simulink model "DFIG_FILTER"  (R2023a)
settings: Solver=ode23t  StartTime=0.0  StopTime=25  MaxStep=1e-6  RelTol=1e-3
model workspace (MAT data in the model file):
  Ts_phasor = 10
undefined symbols (not defined in the file): Base_Power, D1, Delta, F, find_system, Fnom, gcbh, H, ILd_init, ILq_init, Imax_grid_conv, Init, j, Ki_dc_reg, Ki_grid_side_cur_reg, Ki_power_reg, Ki_Q, Ki_rotor_side_cur_reg, Ki_volt_reg, Kp_dc_reg, Kp_grid_side_cur_reg, Kp_power_reg, Kp_Q, Kp_rotor_side_cur_reg, Kp_volt_reg, L_RL, Llr, Lls, p, Pnom, power_A, power_B, power_D, R_RL, Rr, Rs, speed_A, speed_B, speed_C, speed_D, sps_rtmsupport, Vcontrol, Vnom, Wind_On
libraries: spsPower3phPhasorLib x9, spsOnDelayLib x9, spsThreePhaseVIMeasurementLib x8, simulink_extras x5, spsRMSLib x4, spsControlledCurrentSourceLib x4, spsGroundLib x3, spsSeriesRLCBranchLib x2, spsThreePhaseSeriesRLCBranchLib x2, spspowerguiLib x2, spsThreePhasePISectionLineLib x2, spsThreePhaseTransformerTwoWindingsLib x2
(part 2 of 6)

== system DFIG_FILTER/MODEL (PHASER)/Wind turbine Data acquisition2 ==
  Constant : Constant  Value=0
  Gain3 : Gain  Gain=1/3  SaturateOnIntegerOverflow=on  OutDataTypeStr=Inherit: Same as input  ParamDataTypeStr=Inherit: Same as input
  Gain4 : Gain  Gain=1/3  SaturateOnIntegerOverflow=on  OutDataTypeStr=Inherit: Same as input  ParamDataTypeStr=Inherit: Same as input
  MW : Gain  Gain=-1/1e6  SaturateOnIntegerOverflow=on  OutDataTypeStr=Inherit: Same as input  ParamDataTypeStr=Inherit: Same as input
  MW1 : Gain  Gain=-1/1e6  SaturateOnIntegerOverflow=on  OutDataTypeStr=Inherit: Same as input  ParamDataTypeStr=Inherit: Same as input
  Mean Value1 : Subsystem  mask(Mean value){Period=1/60}
      mask prompts: Period "Averaging period (s):"
      mask help: This block uses the running window averaging technique to compute the mean value of the input signal over the specified period.
  Mean Value2 : Subsystem  mask(Mean value){Period=1/60}
      mask prompts: Period "Averaging period (s):"
      mask help: This block uses the running window averaging technique to compute the mean value of the input signal over the specified period.
  "Power (3ph, Phasor)" : spsPower3phPhasorLib/Power (3ph, Phasor)
  Sum : Sum  Inputs=1  InputSameDT=on  SaturateOnIntegerOverflow=on  OutDataTypeStr=Inherit: Same as first input
  Sum1 : Sum  Inputs=1  InputSameDT=on  SaturateOnIntegerOverflow=on  OutDataTypeStr=Inherit: Same as first input
  abc_to_pos : Gain  Gain=[1 exp(j*2*pi/3) exp(-j*2*pi/3)]  SaturateOnIntegerOverflow=on  OutDataTypeStr=Inherit: Same as input  ParamDataTypeStr=Inherit: Same as input
  abc_to_pos1 : Gain  Gain=[1 exp(j*2*pi/3) exp(-j*2*pi/3)]  SaturateOnIntegerOverflow=on  OutDataTypeStr=Inherit: Same as input  ParamDataTypeStr=Inherit: Same as input
  "magnitude positive seq. " : Subsystem
  magnitude positivie seq : Subsystem
  pu->A : Gain  Gain=(6*1.5e6/0.9)/sqrt(3)/575*sqrt(2)  SaturateOnIntegerOverflow=on  OutDataTypeStr=Inherit: Same as input  ParamDataTypeStr=Inherit: Same as input
  pu->V : Gain  Gain=575*sqrt(2)/sqrt(3)  SaturateOnIntegerOverflow=on  OutDataTypeStr=Inherit: Same as input  ParamDataTypeStr=Inherit: Same as input
  Vabc_BFF : Outport  VectorParamsAs1DForOutWhenUnconnected=off
  Iabc_BFF : Outport  Port=2  VectorParamsAs1DForOutWhenUnconnected=off
  P_mean : Outport  Port=3  VectorParamsAs1DForOutWhenUnconnected=off
  Q_mean : Outport  Port=4  VectorParamsAs1DForOutWhenUnconnected=off
  wires:
  [Iabc_BFF] -> abc_to_pos1/1, pu->A/1
  [Vabc_BFF] -> pu->V/1, abc_to_pos/1
  pu->A/1 -> "Power (3ph, Phasor)"/2
  pu->V/1 -> "Power (3ph, Phasor)"/1
  MW/1 -> Mean Value1/1(In)
  MW1/1 -> Mean Value2/1(In)
  "magnitude positive seq. "/1(Out1) -> Iabc_BFF/1
  magnitude positivie seq/1(Out1) -> Vabc_BFF/1
  abc_to_pos/1 -> Sum/1
  Sum/1 -> Gain3/1
  Sum1/1 -> Gain4/1
  Gain3/1 -> magnitude positivie seq/1(In1)
  abc_to_pos1/1 -> Sum1/1
  Gain4/1 -> "magnitude positive seq. "/1(In1)
  Mean Value1/1(Mean) -> P_mean/1
  Mean Value2/1(Mean) -> Q_mean/1
  Constant/1 -> Mean Value1/2(Init), Mean Value2/2(Init)
  "Power (3ph, Phasor)"/1 -> MW/1
  "Power (3ph, Phasor)"/2 -> MW1/1

== system DFIG_FILTER/MODEL (PHASER)/Wind turbine Data acquisition3 ==
  Constant : Constant  Value=0
  Gain3 : Gain  Gain=1/3  SaturateOnIntegerOverflow=on  OutDataTypeStr=Inherit: Same as input  ParamDataTypeStr=Inherit: Same as input
  Gain4 : Gain  Gain=1/3  SaturateOnIntegerOverflow=on  OutDataTypeStr=Inherit: Same as input  ParamDataTypeStr=Inherit: Same as input
  MW : Gain  Gain=-1/1e6  SaturateOnIntegerOverflow=on  OutDataTypeStr=Inherit: Same as input  ParamDataTypeStr=Inherit: Same as input
  MW1 : Gain  Gain=-1/1e6  SaturateOnIntegerOverflow=on  OutDataTypeStr=Inherit: Same as input  ParamDataTypeStr=Inherit: Same as input
  Mean Value1 : Subsystem  mask(Mean value){Period=1/60}
      mask prompts: Period "Averaging period (s):"
      mask help: This block uses the running window averaging technique to compute the mean value of the input signal over the specified period.
  Mean Value2 : Subsystem  mask(Mean value){Period=1/60}
      mask prompts: Period "Averaging period (s):"
      mask help: This block uses the running window averaging technique to compute the mean value of the input signal over the specified period.
  "Power (3ph, Phasor)" : spsPower3phPhasorLib/Power (3ph, Phasor)
  Sum : Sum  Inputs=1  InputSameDT=on  SaturateOnIntegerOverflow=on  OutDataTypeStr=Inherit: Same as first input
  Sum1 : Sum  Inputs=1  InputSameDT=on  SaturateOnIntegerOverflow=on  OutDataTypeStr=Inherit: Same as first input
  abc_to_pos : Gain  Gain=[1 exp(j*2*pi/3) exp(-j*2*pi/3)]  SaturateOnIntegerOverflow=on  OutDataTypeStr=Inherit: Same as input  ParamDataTypeStr=Inherit: Same as input
  abc_to_pos1 : Gain  Gain=[1 exp(j*2*pi/3) exp(-j*2*pi/3)]  SaturateOnIntegerOverflow=on  OutDataTypeStr=Inherit: Same as input  ParamDataTypeStr=Inherit: Same as input
  "magnitude positive seq. " : Subsystem
  magnitude positivie seq : Subsystem
  pu->A : Gain  Gain=(6*1.5e6/0.9)/sqrt(3)/575*sqrt(2)  SaturateOnIntegerOverflow=on  OutDataTypeStr=Inherit: Same as input  ParamDataTypeStr=Inherit: Same as input
  pu->V : Gain  Gain=575*sqrt(2)/sqrt(3)  SaturateOnIntegerOverflow=on  OutDataTypeStr=Inherit: Same as input  ParamDataTypeStr=Inherit: Same as input
  Vabc_BFF : Outport  VectorParamsAs1DForOutWhenUnconnected=off
  Iabc_BFF : Outport  Port=2  VectorParamsAs1DForOutWhenUnconnected=off
  P_mean : Outport  Port=3  VectorParamsAs1DForOutWhenUnconnected=off
  Q_mean : Outport  Port=4  VectorParamsAs1DForOutWhenUnconnected=off
  wires:
  [Iabc_BFF] -> abc_to_pos1/1, pu->A/1
  [Vabc_BFF] -> pu->V/1, abc_to_pos/1
  pu->A/1 -> "Power (3ph, Phasor)"/2
  pu->V/1 -> "Power (3ph, Phasor)"/1
  MW/1 -> Mean Value1/1(In)
  MW1/1 -> Mean Value2/1(In)
  "magnitude positive seq. "/1(Out1) -> Iabc_BFF/1
  magnitude positivie seq/1(Out1) -> Vabc_BFF/1
  abc_to_pos/1 -> Sum/1
  Sum/1 -> Gain3/1
  Sum1/1 -> Gain4/1
  Gain3/1 -> magnitude positivie seq/1(In1)
  abc_to_pos1/1 -> Sum1/1
  Gain4/1 -> "magnitude positive seq. "/1(In1)
  Mean Value1/1(Mean) -> P_mean/1
  Mean Value2/1(Mean) -> Q_mean/1
  Constant/1 -> Mean Value1/2(Init), Mean Value2/2(Init)
  "Power (3ph, Phasor)"/1 -> MW/1
  "Power (3ph, Phasor)"/2 -> MW1/1

== system DFIG_FILTER/MODEL (PHASER)/Wind turbine Data acquisition4 ==
  Constant : Constant  Value=0
  Gain3 : Gain  Gain=1/3  SaturateOnIntegerOverflow=on  OutDataTypeStr=Inherit: Same as input  ParamDataTypeStr=Inherit: Same as input
  Gain4 : Gain  Gain=1/3  SaturateOnIntegerOverflow=on  OutDataTypeStr=Inherit: Same as input  ParamDataTypeStr=Inherit: Same as input
  MW : Gain  Gain=-1/1e6  SaturateOnIntegerOverflow=on  OutDataTypeStr=Inherit: Same as input  ParamDataTypeStr=Inherit: Same as input
  MW1 : Gain  Gain=-1/1e6  SaturateOnIntegerOverflow=on  OutDataTypeStr=Inherit: Same as input  ParamDataTypeStr=Inherit: Same as input
  Mean Value1 : Subsystem  mask(Mean value){Period=1/60}
      mask prompts: Period "Averaging period (s):"
      mask help: This block uses the running window averaging technique to compute the mean value of the input signal over the specified period.
  Mean Value2 : Subsystem  mask(Mean value){Period=1/60}
      mask prompts: Period "Averaging period (s):"
      mask help: This block uses the running window averaging technique to compute the mean value of the input signal over the specified period.
  "Power (3ph, Phasor)" : spsPower3phPhasorLib/Power (3ph, Phasor)
  Sum : Sum  Inputs=1  InputSameDT=on  SaturateOnIntegerOverflow=on  OutDataTypeStr=Inherit: Same as first input
  Sum1 : Sum  Inputs=1  InputSameDT=on  SaturateOnIntegerOverflow=on  OutDataTypeStr=Inherit: Same as first input
  abc_to_pos : Gain  Gain=[1 exp(j*2*pi/3) exp(-j*2*pi/3)]  SaturateOnIntegerOverflow=on  OutDataTypeStr=Inherit: Same as input  ParamDataTypeStr=Inherit: Same as input
  abc_to_pos1 : Gain  Gain=[1 exp(j*2*pi/3) exp(-j*2*pi/3)]  SaturateOnIntegerOverflow=on  OutDataTypeStr=Inherit: Same as input  ParamDataTypeStr=Inherit: Same as input
  "magnitude positive seq. " : Subsystem
  magnitude positivie seq : Subsystem
  pu->A : Gain  Gain=(6*1.5e6/0.9)/sqrt(3)/575*sqrt(2)  SaturateOnIntegerOverflow=on  OutDataTypeStr=Inherit: Same as input  ParamDataTypeStr=Inherit: Same as input
  pu->V : Gain  Gain=575*sqrt(2)/sqrt(3)  SaturateOnIntegerOverflow=on  OutDataTypeStr=Inherit: Same as input  ParamDataTypeStr=Inherit: Same as input
  Vabc_BAF : Outport  VectorParamsAs1DForOutWhenUnconnected=off
  Iabc_BAF : Outport  Port=2  VectorParamsAs1DForOutWhenUnconnected=off
  P_mean : Outport  Port=3  VectorParamsAs1DForOutWhenUnconnected=off
  Q_mean : Outport  Port=4  VectorParamsAs1DForOutWhenUnconnected=off
  wires:
  [Iabc_BAF] -> abc_to_pos1/1, pu->A/1
  [Vabc_BAF] -> pu->V/1, abc_to_pos/1
  pu->A/1 -> "Power (3ph, Phasor)"/2
  pu->V/1 -> "Power (3ph, Phasor)"/1
  MW/1 -> Mean Value1/1(In)
  MW1/1 -> Mean Value2/1(In)
  "magnitude positive seq. "/1(Out1) -> Iabc_BAF/1
  magnitude positivie seq/1(Out1) -> Vabc_BAF/1
  abc_to_pos/1 -> Sum/1
  Sum/1 -> Gain3/1
  Sum1/1 -> Gain4/1
  Gain3/1 -> magnitude positivie seq/1(In1)
  abc_to_pos1/1 -> Sum1/1
  Gain4/1 -> "magnitude positive seq. "/1(In1)
  Mean Value1/1(Mean) -> P_mean/1
  Mean Value2/1(Mean) -> Q_mean/1
  Constant/1 -> Mean Value1/2(Init), Mean Value2/2(Init)
  "Power (3ph, Phasor)"/1 -> MW/1
  "Power (3ph, Phasor)"/2 -> MW1/1

== system DFIG_FILTER/MODEL (PHASER)/Wind turbine Data acquisition5 ==
  Constant : Constant  Value=0
  Gain3 : Gain  Gain=1/3  SaturateOnIntegerOverflow=on  OutDataTypeStr=Inherit: Same as input  ParamDataTypeStr=Inherit: Same as input
  Gain4 : Gain  Gain=1/3  SaturateOnIntegerOverflow=on  OutDataTypeStr=Inherit: Same as input  ParamDataTypeStr=Inherit: Same as input
  MW : Gain  Gain=-1/1e6  SaturateOnIntegerOverflow=on  OutDataTypeStr=Inherit: Same as input  ParamDataTypeStr=Inherit: Same as input
  MW1 : Gain  Gain=-1/1e6  SaturateOnIntegerOverflow=on  OutDataTypeStr=Inherit: Same as input  ParamDataTypeStr=Inherit: Same as input
  Mean Value1 : Subsystem  mask(Mean value){Period=1/60}
      mask prompts: Period "Averaging period (s):"
      mask help: This block uses the running window averaging technique to compute the mean value of the input signal over the specified period.
  Mean Value2 : Subsystem  mask(Mean value){Period=1/60}
      mask prompts: Period "Averaging period (s):"
      mask help: This block uses the running window averaging technique to compute the mean value of the input signal over the specified period.
  "Power (3ph, Phasor)" : spsPower3phPhasorLib/Power (3ph, Phasor)
  Sum : Sum  Inputs=1  InputSameDT=on  SaturateOnIntegerOverflow=on  OutDataTypeStr=Inherit: Same as first input
  Sum1 : Sum  Inputs=1  InputSameDT=on  SaturateOnIntegerOverflow=on  OutDataTypeStr=Inherit: Same as first input
  abc_to_pos : Gain  Gain=[1 exp(j*2*pi/3) exp(-j*2*pi/3)]  SaturateOnIntegerOverflow=on  OutDataTypeStr=Inherit: Same as input  ParamDataTypeStr=Inherit: Same as input
  abc_to_pos1 : Gain  Gain=[1 exp(j*2*pi/3) exp(-j*2*pi/3)]  SaturateOnIntegerOverflow=on  OutDataTypeStr=Inherit: Same as input  ParamDataTypeStr=Inherit: Same as input
  "magnitude positive seq. " : Subsystem
  magnitude positivie seq : Subsystem
  pu->A : Gain  Gain=(6*1.5e6/0.9)/sqrt(3)/575*sqrt(2)  SaturateOnIntegerOverflow=on  OutDataTypeStr=Inherit: Same as input  ParamDataTypeStr=Inherit: Same as input
  pu->V : Gain  Gain=575*sqrt(2)/sqrt(3)  SaturateOnIntegerOverflow=on  OutDataTypeStr=Inherit: Same as input  ParamDataTypeStr=Inherit: Same as input
  Vabc_BAF : Outport  VectorParamsAs1DForOutWhenUnconnected=off
  Iabc_BAF : Outport  Port=2  VectorParamsAs1DForOutWhenUnconnected=off
  P_mean : Outport  Port=3  VectorParamsAs1DForOutWhenUnconnected=off
  Q_mean : Outport  Port=4  VectorParamsAs1DForOutWhenUnconnected=off
  wires:
  [Vabc_B575] -> abc_to_pos1/1, pu->A/1
  [Vabc_B575] -> pu->V/1, abc_to_pos/1
  pu->A/1 -> "Power (3ph, Phasor)"/2
  pu->V/1 -> "Power (3ph, Phasor)"/1
  MW/1 -> Mean Value1/1(In)
  MW1/1 -> Mean Value2/1(In)
  "magnitude positive seq. "/1(Out1) -> Iabc_BAF/1
  magnitude positivie seq/1(Out1) -> Vabc_BAF/1
  abc_to_pos/1 -> Sum/1
  Sum/1 -> Gain3/1
  Sum1/1 -> Gain4/1
  Gain3/1 -> magnitude positivie seq/1(In1)
  abc_to_pos1/1 -> Sum1/1
  Gain4/1 -> "magnitude positive seq. "/1(In1)
  Mean Value1/1(Mean) -> P_mean/1
  Mean Value2/1(Mean) -> Q_mean/1
  Constant/1 -> Mean Value1/2(Init), Mean Value2/2(Init)
  "Power (3ph, Phasor)"/1 -> MW/1
  "Power (3ph, Phasor)"/2 -> MW1/1

== system DFIG_FILTER/FILTER (DISCRETE) /controller1/WMPID ==
  In1 : Inport  PortDimensions=3
  Cast To Double : DataTypeConversion  OutDataTypeStr=double  SaturateOnIntegerOverflow=off  RndMeth=Floor
  Cast To Double1 : DataTypeConversion  OutDataTypeStr=double  SaturateOnIntegerOverflow=off  RndMeth=Floor
  Derivative : Derivative
  Integrator : Integrator
  Kd : Gain
  Ke : Gain
  Ki : Gain  Gain=2
  Kp : Gain  Gain=25
  Product1 : Product
  Sum7 : Sum  Inputs=|+++
  Sum8 : Sum  Inputs=|++
  Out1 : Outport  PortDimensions=3
  wires:
  In1/1 -> Kp/1, Product1/2, Product1/1, Derivative/1, Ki/1
  Sum8/1 -> Out1/1
  Integrator/1 -> Sum7/2
  Derivative/1 -> Kd/1
  Product1/1 -> Ke/1
  Kd/1 -> Sum7/3
  Ki/1 -> Integrator/1
  Kp/1 -> Sum7/1
  Ke/1 -> Cast To Double/1
  Cast To Double/1 -> Sum8/1
  Sum7/1 -> Cast To Double1/1
  Cast To Double1/1 -> Sum8/2

== system DFIG_FILTER/MODEL (PHASER)/Grid Data acquisition/Mean Value1 ==
  note: Mean value
  In : Inport
  Init : Inport  Port=2
  Gain : Gain  Gain=1/Period  SaturateOnIntegerOverflow=on  OutDataTypeStr=Inherit: Same as input  ParamDataTypeStr=Inherit: Same as input
  Step : Step  Time=Period+eps  SampleTime=0
  Sum : Sum  Inputs=+-  InputSameDT=on  SaturateOnIntegerOverflow=on  OutDataTypeStr=Inherit: Same as first input
  Switch : Switch  Threshold=0.5  InputSameDT=off
  Transport Delay : TransportDelay  DelayTime=Period
  integrator : Integrator
  Mean : Outport  VectorParamsAs1DForOutWhenUnconnected=off
  wires:
  Transport Delay/1 -> Sum/2
  integrator/1 -> Transport Delay/1, Sum/1
  In/1 -> integrator/1
  Sum/1 -> Gain/1
  Gain/1 -> Switch/1
  Switch/1 -> Mean/1
  Step/1 -> Switch/2
  Init/1 -> Switch/3

== system DFIG_FILTER/MODEL (PHASER)/Grid Data acquisition/Mean Value2 ==
  note: Mean value
  In : Inport
  Init : Inport  Port=2
  Gain : Gain  Gain=1/Period  SaturateOnIntegerOverflow=on  OutDataTypeStr=Inherit: Same as input  ParamDataTypeStr=Inherit: Same as input
  Step : Step  Time=Period+eps  SampleTime=0
  Sum : Sum  Inputs=+-  InputSameDT=on  SaturateOnIntegerOverflow=on  OutDataTypeStr=Inherit: Same as first input
  Switch : Switch  Threshold=0.5  InputSameDT=off
  Transport Delay : TransportDelay  DelayTime=Period
  integrator : Integrator
  Mean : Outport  VectorParamsAs1DForOutWhenUnconnected=off
  wires:
  Init/1 -> Switch/3
  Step/1 -> Switch/2
  Switch/1 -> Mean/1
  Gain/1 -> Switch/1
  Sum/1 -> Gain/1
  In/1 -> integrator/1
  integrator/1 -> Sum/1, Transport Delay/1
  Transport Delay/1 -> Sum/2

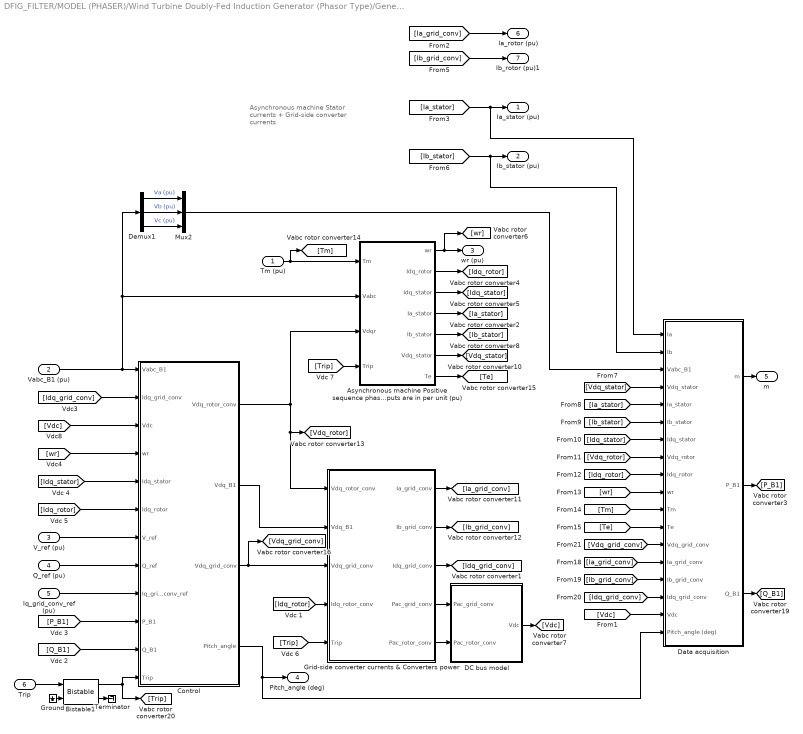
== system DFIG_FILTER/MODEL (PHASER)/Wind Turbine Doubly-Fed Induction Generator (Phasor Type)/Generator & Converters ==
  note: Asynchronous machine
      | Stator currents
      | +
      | Grid-side converter
      | currents
  Tm (pu) : Inport
  Vabc_B1 (pu) : Inport  Port=2
  V_ref (pu) : Inport  Port=3
  Q_ref (pu) : Inport  Port=4
  Iq_grid_conv_ref (pu) : Inport  Port=5
  Trip : Inport  Port=6
  Asynchronous machine Positive sequence phasor model Inputs and outputs are in per unit (pu) : Subsystem  mask(Asynchronous Machine Model){nom=[ Pnom Vnom Fnom ], sta=[ Rs Lls], rot=[ Rr Llr], Lm=Lm, mec=[H F p], ini=init}
      mask prompts: nom "Nom. power,L-L volt. and freq. [ Pn(VA),Vn(Vrms),fn(Hz) ]:"; sta "Stator [ Rs,Lls (pu) ]:"; rot "Rotor [ Rr',Llr' (pu) ]:"; Lm "Magnetizing inductance Lm (pu):"; mec "Inertia constant,friction factor and pairs of poles [ H(s)  F(pu)  p() ]:"; ini "Initial conditions [s()  th(deg)  Is(pu)  ph_Is(deg)  Ir(pu)  ph_Ir(deg)]:"
      mask help: Implements a three-phase asynchronous machine (wound rotor) modelled in the dq stator reference frame. Stator and rotor windings are connected in wye to an internal neutral point.
      mask init:
      | %Initializes the Asynchronous Machine block before simulation.
      | 
      | % Base angular frequency
      | web=nom(3)*2*pi;
      | 
      | Rs=sta(1); Lls=sta(2);		% stator resistance and leakage inductance
      | Rr=rot(1); Llr=rot(2);		% rotor resistance and leakage inductance
      | Lm=Lm(1);			        % mutual inductance
      | H=mec(1); F=mec(2); p=mec(3);	% inertia, friction and pole pairs
      | s=ini(1);			% initial slip
      | wmo=1-s;			% initial speed
      | tho=ini(2)*pi/180;		% initial rotor angle
      | 
      | iso_mag=ini(3); iso_ph=ini(4)*pi/180; % init. stator current, phase A
      | iro_mag=ini(5); iro_ph=ini(6)*pi/180; % init. rotor current, phase A
      | 
      | % conversion of initial stator and rotor currents from polar to rectangular
      | % coordinates
      | [isdo,isqo]=pol2cart(iso_ph,iso_mag);
      | [irdo,irqo]=pol2cart(iro_ph,iro_mag);
      | 
      | % Initial fluxes (pu): inductances in pu, currents in pu
      | phisqo=((Lls+Lm)*isqo+Lm*irqo);
      | phisdo=((Lls+Lm)*isdo+Lm*irdo);
      | phirqo=((Llr+Lm)*irqo+Lm*isqo);
      | phirdo=((Llr+Lm)*irdo+Lm*isdo);
      | 
      | % Other inductances -------------------------------------------------------
      | 
      | Laq=1/(1/Lm+1/Lls+1/Llr);
      | Lad=Laq;
      mask Help: First 3 inputs: Stator terminals = phases a, b and c; 4th input: Simulink signal = Mechanical torque applied to the shaft (pu, >0 for motor mode, <0 for generator mode); First 3 outputs: Rotor terminals = phases a, b and c; 4th output: Simulink measurement output = vector (20x1) containing the following (all currents flowing into the machine): [1-3] : Rotor line currents ira, irb and irc; [4-5] : Rotor currents iqr and idr; [6-7] : Rotor fluxes phiqr and  phidr; [8-9] : Rotor voltages vqr and vdr; [10-12] : Stator line currents isa, isb, isc; [13-14] : Stator currents iqs and ids; [15-16] : Stator fluxes phiqs and  phids; [17-18] : Stator voltages vqs and vds; [19] : Rotor speed wm; [20 ]: Electromagnetic torque Te. Units of output measurement depend on checkbox in block's dialog box.
  Bistable1 : spsBistableLib/Bistable  Qpriority=Set  ic=0  Ts=0
      settings: LibrarySourceBlock=sps_lib/Control/Bistable
  Control : Subsystem
  DC bus model : Subsystem  mask(DC bus model){Pnom=Pnom, C=capacitor, Vdc_Init=Vdc_nom}
      mask prompts: Pnom "Nominal power (W):"; C "Capacitor (F):"; Vdc_Init "Initial voltage (V):"
  Data acquisition : Subsystem
  Demux1 : Demux  Outputs=3
      settings: DisplayOption=none
  Grid-side converter currents & Converters power : Subsystem
  Ground : Ground
  Mux2 : Mux  Inputs=3
  Terminator : Terminator
  Ia_stator (pu) : Outport  VectorParamsAs1DForOutWhenUnconnected=off
  Ib_stator (pu) : Outport  Port=2  VectorParamsAs1DForOutWhenUnconnected=off
  wr (pu) : Outport  Port=3  VectorParamsAs1DForOutWhenUnconnected=off
  Pitch_angle (deg) : Outport  Port=4  VectorParamsAs1DForOutWhenUnconnected=off
  m : Outport  Port=5  VectorParamsAs1DForOutWhenUnconnected=off
  Ia_rotor (pu) : Outport  Port=6  VectorParamsAs1DForOutWhenUnconnected=off
  Ib_rotor (pu)1 : Outport  Port=7  VectorParamsAs1DForOutWhenUnconnected=off
  wires:
  DC bus model/1(Vdc) -> [Vdc]
  [Idq_rotor] -> Control/6(Idq_rotor)
  [Idq_stator] -> Control/5(Idq_stator)
  [Vdc] -> Control/3(Vdc)
  [wr] -> Control/4(wr)
  Control/3(Vdq_grid_conv) -> Grid-side converter currents & Converters power/3(Vdq_grid_conv), [Vdq_grid_conv]
  Control/1(Vdq_rotor_conv) -> Asynchronous machine Positive sequence phasor model Inputs and outputs are in per unit (pu)/3("Vdqr "), Grid-side converter currents & Converters power/1(Vdq_rotor_conv), [Vdq_rotor]
  Control/2(Vdq_B1) -> Grid-side converter currents & Converters power/2(Vdq_B1)
  Grid-side converter currents & Converters power/3(Idq_grid_conv) -> [Idq_grid_conv]
  [Idq_grid_conv] -> Control/2(Idq_grid_conv)
  Asynchronous machine Positive sequence phasor model Inputs and outputs are in per unit (pu)/3(Idq_stator) -> [Idq_stator]
  Asynchronous machine Positive sequence phasor model Inputs and outputs are in per unit (pu)/2(Idq_rotor) -> [Idq_rotor]
  Tm (pu)/1 -> Asynchronous machine Positive sequence phasor model Inputs and outputs are in per unit (pu)/1(Tm), [Tm]
  Asynchronous machine Positive sequence phasor model Inputs and outputs are in per unit (pu)/5(Ib_stator) -> [Ib_stator]
  Asynchronous machine Positive sequence phasor model Inputs and outputs are in per unit (pu)/4(Ia_stator) -> [Ia_stator]
  [Idq_rotor] -> Grid-side converter currents & Converters power/4(Idq_rotor_conv)
  Grid-side converter currents & Converters power/4(Pac_grid_conv) -> DC bus model/1(Pac_grid_conv)
  Grid-side converter currents & Converters power/5(Pac_rotor_conv) -> DC bus model/2(Pac_rotor_conv)
  Vabc_B1 (pu)/1 -> Control/1(Vabc_B1), Asynchronous machine Positive sequence phasor model Inputs and outputs are in per unit (pu)/2(Vabc), Demux1/1
  [Ia_stator] -> Ia_stator (pu)/1, Data acquisition/1(Ia)
  [Ib_stator] -> Ib_stator (pu)/1, Data acquisition/2(Ib)
  Asynchronous machine Positive sequence phasor model Inputs and outputs are in per unit (pu)/1(wr) -> wr (pu)/1, [wr]
  Asynchronous machine Positive sequence phasor model Inputs and outputs are in per unit (pu)/6(Vdq_stator) -> [Vdq_stator]
  Grid-side converter currents & Converters power/1(Ia_grid_conv) -> [Ia_grid_conv]
  Grid-side converter currents & Converters power/2(Ib_grid_conv) -> [Ib_grid_conv]
  [Ia_grid_conv] -> Ia_rotor (pu)/1
  [Ib_grid_conv] -> Ib_rotor (pu)1/1
  Asynchronous machine Positive sequence phasor model Inputs and outputs are in per unit (pu)/7(Te) -> [Te]
  [Idq_grid_conv] -> Data acquisition/16(Idq_grid_conv)
  [Ib_grid_conv] -> Data acquisition/15(Ib_grid_conv)
  [Ia_grid_conv] -> Data acquisition/14(Ia_grid_conv)
  [Vdq_grid_conv] -> Data acquisition/13(Vdq_grid_conv)
  [Te] -> Data acquisition/12(Te)
  [Tm] -> Data acquisition/11(Tm)
  [wr] -> Data acquisition/10(wr)
  [Idq_rotor] -> Data acquisition/9(Idq_rotor)
  [Vdq_rotor] -> Data acquisition/8(Vdq_rotor)
  [Idq_stator] -> Data acquisition/7(Idq_stator)
  [Ib_stator] -> Data acquisition/6(Ib_stator)
  [Ia_stator] -> Data acquisition/5(Ia_stator)
  [Vdq_stator] -> Data acquisition/4(Vdq_stator)
  Data acquisition/1(m) -> m/1
  [Vdc] -> Data acquisition/17(Vdc)
  Demux1/1 -> Mux2/1  "Va (pu)"
  Demux1/2 -> Mux2/2  "Vb (pu)"
  Mux2/1 -> Data acquisition/3(Vabc_B1)
  Demux1/3 -> Mux2/3  "Vc (pu)"
  Data acquisition/3(Q_B1) -> [Q_B1]
  Q_ref (pu)/1 -> Control/8(Q_ref)
  Iq_grid_conv_ref (pu)/1 -> Control/9(Iq_grid_conv_ref)
  Data acquisition/2(P_B1) -> [P_B1]
  [P_B1] -> Control/10(P_B1)
  [Q_B1] -> Control/11(Q_B1)
  V_ref (pu)/1 -> Control/7(V_ref)
  [Trip] -> Grid-side converter currents & Converters power/5(Trip)
  [Trip] -> Asynchronous machine Positive sequence phasor model Inputs and outputs are in per unit (pu)/4(Trip)
  Trip/1 -> Bistable1/1
  Bistable1/2 -> Terminator/1
  Ground/1 -> Bistable1/2
  Bistable1/1 -> [Trip], Control/12(Trip)
  Control/4(Pitch_angle) -> Data acquisition/18(Pitch_angle (deg)), Pitch_angle (deg)/1

== system DFIG_FILTER/MODEL (PHASER)/Wind Turbine Protection/Protection System ==
  Vabc (pu) : Inport  PortDimensions=3
  Iabc (pu) : Inport  Port=2  PortDimensions=3
  Vdc (V) : Inport  Port=3  PortDimensions=1
  Reset : Inport  Port=4  PortDimensions=1
  Speed (pu) : Inport  Port=5  PortDimensions=1
  AC Current Protection : Subsystem
  AC Voltage Protection : Subsystem
  Bistable1 : spsBistableLib/Bistable  Qpriority=Set  ic=0  Ts=0
  Clock : Clock
  Constant : Constant  Value=Delay_Protection
  DC Voltage Protection : Subsystem
  Decoding : Subsystem
  Encoding : Subsystem
  Logical Operator : Logic  Operator=OR  Inputs=10  AllPortsSameDT=off
  Logical Operator1 : Logic  AllPortsSameDT=off
  Logical Operator2 : Logic  Operator=NOT  AllPortsSameDT=off
  Logical Operator3 : Logic  AllPortsSameDT=off
  Memory : Memory  InheritSampleTime=on
  Memory1 : Memory  InheritSampleTime=on
  Monostable1 : spsMonostableLib/Monostable  EdgeDetect=Rising  PulseDuration=1e-9  ic=0  Ts=0
  Relational Operator10 : RelationalOperator  InputSameDT=off
  Sample & Hold : Subsystem  DialogController=POWERSYS.PowerSysDialog  mask(Sample & Hold){ic=0}
      mask prompts: ic "Initial condition:"
      mask help: The output follows input 1 (In) as long as input 2 (S) is TRUE (1) . The output is held when input 2 becomes FALSE (0). The output initial value is specified by the parameter "Initial condition".
      mask init:
      | power_initmask();
      mask Help: This block is part of a subset of blocks in the Extras library that does not have documentation associated with it, other than the block mask description.
      mask Display: disp('S/H')
  Sample & Hold1 : Subsystem  DialogController=POWERSYS.PowerSysDialog  mask(Sample & Hold){ic=0}
      mask prompts: ic "Initial condition:"
      mask help: The output follows input 1 (In) as long as input 2 (S) is TRUE (1) . The output is held when input 2 becomes FALSE (0). The output initial value is specified by the parameter "Initial condition".
      mask init:
      | power_initmask();
      mask Help: This block is part of a subset of blocks in the Extras library that does not have documentation associated with it, other than the block mask description.
      mask Display: disp('S/H')
  Terminator : Terminator
  Under/Over Speed Protection : Subsystem
  Trip : Outport  VectorParamsAs1DForOutWhenUnconnected=off
  TripTime : Outport  Port=2  VectorParamsAs1DForOutWhenUnconnected=off
  TripStatus : Outport  Port=3  VectorParamsAs1DForOutWhenUnconnected=off
  wires:
  Speed (pu)/1 -> Under/Over Speed Protection/1(Speed)
  Under/Over Speed Protection/2(MaxSpeed) -> Encoding/10(In10), Logical Operator/10
  Under/Over Speed Protection/1(MinSpeed) -> Encoding/9(In9), Logical Operator/9
  Relational Operator10/1 -> Logical Operator1/2
  Logical Operator/1 -> Logical Operator1/1
  Clock/1 -> Sample & Hold1/1(In), Relational Operator10/1
  Constant/1 -> Relational Operator10/2
  Monostable1/1 -> Sample & Hold1/2(S), Sample & Hold/2(S)
  Sample & Hold1/1("   ") -> TripTime/1
  AC Voltage Protection/4(MaxV0V1) -> Encoding/7(In7), Logical Operator/7
  AC Voltage Protection/3(MaxV2V1) -> Encoding/6(In6), Logical Operator/6
  AC Voltage Protection/2(MaxV1) -> Encoding/5(In5), Logical Operator/5
  AC Voltage Protection/1(MinV1) -> Encoding/4(In4), Logical Operator/4
  AC Current Protection/3(MaxI2I1) -> Encoding/3(In3), Logical Operator/3
  AC Current Protection/2(MaxI1) -> Encoding/2(In2), Logical Operator/2
  AC Current Protection/1(MaxIinst) -> Encoding/1(In1), Logical Operator/1
  Vabc (pu)/1 -> AC Voltage Protection/1(abc)
  Iabc (pu)/1 -> AC Current Protection/1(abc)
  Decoding/1(Out) -> TripStatus/1
  Sample & Hold/1("   ") -> Decoding/1(Code)
  Bistable1/2 -> Terminator/1
  Memory/1 -> Monostable1/1, Memory1/1
  Bistable1/1 -> Memory/1
  Encoding/1(Code) -> Sample & Hold/1(In)
  Logical Operator1/1 -> Bistable1/1, Logical Operator2/1
  Logical Operator3/1 -> Bistable1/2
  Reset/1 -> Logical Operator3/2
  Logical Operator2/1 -> Logical Operator3/1
  DC Voltage Protection/1(MaxVdc) -> Encoding/8(In8), Logical Operator/8
  Vdc (V)/1 -> DC Voltage Protection/1(Vdc)
  Memory1/1 -> Trip/1

== system DFIG_FILTER/MODEL (PHASER)/Wind turbine Data acquisition/Mean Value1 ==
  note: Mean value
  In : Inport
  Init : Inport  Port=2
  Gain : Gain  Gain=1/Period  SaturateOnIntegerOverflow=on  OutDataTypeStr=Inherit: Same as input  ParamDataTypeStr=Inherit: Same as input
  Step : Step  Time=Period+eps  SampleTime=0
  Sum : Sum  Inputs=+-  InputSameDT=on  SaturateOnIntegerOverflow=on  OutDataTypeStr=Inherit: Same as first input
  Switch : Switch  Threshold=0.5  InputSameDT=off
  Transport Delay : TransportDelay  DelayTime=Period
  integrator : Integrator
  Mean : Outport  VectorParamsAs1DForOutWhenUnconnected=off
  wires:
  Transport Delay/1 -> Sum/2
  integrator/1 -> Transport Delay/1, Sum/1
  In/1 -> integrator/1
  Sum/1 -> Gain/1
  Gain/1 -> Switch/1
  Switch/1 -> Mean/1
  Step/1 -> Switch/2
  Init/1 -> Switch/3

== system DFIG_FILTER/MODEL (PHASER)/Wind turbine Data acquisition/Mean Value2 ==
  note: Mean value
  In : Inport
  Init : Inport  Port=2
  Gain : Gain  Gain=1/Period  SaturateOnIntegerOverflow=on  OutDataTypeStr=Inherit: Same as input  ParamDataTypeStr=Inherit: Same as input
  Step : Step  Time=Period+eps  SampleTime=0
  Sum : Sum  Inputs=+-  InputSameDT=on  SaturateOnIntegerOverflow=on  OutDataTypeStr=Inherit: Same as first input
  Switch : Switch  Threshold=0.5  InputSameDT=off
  Transport Delay : TransportDelay  DelayTime=Period
  integrator : Integrator
  Mean : Outport  VectorParamsAs1DForOutWhenUnconnected=off
  wires:
  Init/1 -> Switch/3
  Step/1 -> Switch/2
  Switch/1 -> Mean/1
  Gain/1 -> Switch/1
  Sum/1 -> Gain/1
  In/1 -> integrator/1
  integrator/1 -> Sum/1, Transport Delay/1
  Transport Delay/1 -> Sum/2

== system DFIG_FILTER/MODEL (PHASER)/Wind turbine Data acquisition/magnitude positive seq.  ==
  In1 : Inport
  Complex to Real-Imag : ComplexToRealImag
  Fourier1 : Subsystem  mask(Fourier analyser){f1=60, n=0}
      mask prompts: f1 "Fundamental frequency f1 (Hz):"; n "Harmonic n (0=DC; 1=fundamental; 2=2nd harm;  ...) :"
      mask help: The Fourier block performs a Fourier analysis of the input signal over a running window of one cycle of the fundamental frequency. First and second outputs return respectively the magnitude and phase (degrees) of the harmonic component specified.
      mask init:
      | k=2-(n==0);
      mask Help: helpview(psbhelp)
  Fourier2 : Subsystem  mask(Fourier analyser){f1=60, n=0}
      mask prompts: f1 "Fundamental frequency f1 (Hz):"; n "Harmonic n (0=DC; 1=fundamental; 2=2nd harm;  ...) :"
      mask help: The Fourier block performs a Fourier analysis of the input signal over a running window of one cycle of the fundamental frequency. First and second outputs return respectively the magnitude and phase (degrees) of the harmonic component specified.
      mask init:
      | k=2-(n==0);
      mask Help: helpview(psbhelp)
  Math Function : Math  Operator=hypot  SignedPower=on
  Terminator : Terminator
  Terminator1 : Terminator
  Out1 : Outport  VectorParamsAs1DForOutWhenUnconnected=off
  wires:
  In1/1 -> Complex to Real-Imag/1
  Math Function/1 -> Out1/1
  Fourier2/1(magnitude) -> Math Function/2
  Fourier1/1(magnitude) -> Math Function/1
  Fourier2/2(angle) -> Terminator1/1
  Fourier1/2(angle) -> Terminator/1
  Complex to Real-Imag/2 -> Fourier2/1(signal)
  Complex to Real-Imag/1 -> Fourier1/1(signal)

== system DFIG_FILTER/MODEL (PHASER)/Wind turbine Data acquisition/magnitude positivie seq ==
  In1 : Inport
  Complex to Real-Imag : ComplexToRealImag
  Fourier1 : Subsystem  mask(Fourier analyser){f1=60, n=0}
      mask prompts: f1 "Fundamental frequency f1 (Hz):"; n "Harmonic n (0=DC; 1=fundamental; 2=2nd harm;  ...) :"
      mask help: The Fourier block performs a Fourier analysis of the input signal over a running window of one cycle of the fundamental frequency. First and second outputs return respectively the magnitude and phase (degrees) of the harmonic component specified.
      mask init:
      | k=2-(n==0);
      mask Help: helpview(psbhelp)
  Fourier2 : Subsystem  mask(Fourier analyser){f1=60, n=0}
      mask prompts: f1 "Fundamental frequency f1 (Hz):"; n "Harmonic n (0=DC; 1=fundamental; 2=2nd harm;  ...) :"
      mask help: The Fourier block performs a Fourier analysis of the input signal over a running window of one cycle of the fundamental frequency. First and second outputs return respectively the magnitude and phase (degrees) of the harmonic component specified.
      mask init:
      | k=2-(n==0);
      mask Help: helpview(psbhelp)
  Math Function : Math  Operator=hypot  SignedPower=on
  Terminator : Terminator
  Terminator1 : Terminator
  Out1 : Outport  VectorParamsAs1DForOutWhenUnconnected=off
  wires:
  Complex to Real-Imag/1 -> Fourier1/1(signal)
  Complex to Real-Imag/2 -> Fourier2/1(signal)
  Fourier1/2(angle) -> Terminator/1
  Fourier2/2(angle) -> Terminator1/1
  Fourier1/1(magnitude) -> Math Function/1
  Fourier2/1(magnitude) -> Math Function/2
  Math Function/1 -> Out1/1
  In1/1 -> Complex to Real-Imag/1

== system DFIG_FILTER/MODEL (PHASER)/Wind turbine Data acquisition1/Mean Value1 ==
  note: Mean value
  In : Inport
  Init : Inport  Port=2
  Gain : Gain  Gain=1/Period  SaturateOnIntegerOverflow=on  OutDataTypeStr=Inherit: Same as input  ParamDataTypeStr=Inherit: Same as input
  Step : Step  Time=Period+eps  SampleTime=0
  Sum : Sum  Inputs=+-  InputSameDT=on  SaturateOnIntegerOverflow=on  OutDataTypeStr=Inherit: Same as first input
  Switch : Switch  Threshold=0.5  InputSameDT=off
  Transport Delay : TransportDelay  DelayTime=Period
  integrator : Integrator
  Mean : Outport  VectorParamsAs1DForOutWhenUnconnected=off
  wires:
  Transport Delay/1 -> Sum/2
  integrator/1 -> Transport Delay/1, Sum/1
  In/1 -> integrator/1
  Sum/1 -> Gain/1
  Gain/1 -> Switch/1
  Switch/1 -> Mean/1
  Step/1 -> Switch/2
  Init/1 -> Switch/3

== system DFIG_FILTER/MODEL (PHASER)/Wind turbine Data acquisition1/Mean Value2 ==
  note: Mean value
  In : Inport
  Init : Inport  Port=2
  Gain : Gain  Gain=1/Period  SaturateOnIntegerOverflow=on  OutDataTypeStr=Inherit: Same as input  ParamDataTypeStr=Inherit: Same as input
  Step : Step  Time=Period+eps  SampleTime=0
  Sum : Sum  Inputs=+-  InputSameDT=on  SaturateOnIntegerOverflow=on  OutDataTypeStr=Inherit: Same as first input
  Switch : Switch  Threshold=0.5  InputSameDT=off
  Transport Delay : TransportDelay  DelayTime=Period
  integrator : Integrator
  Mean : Outport  VectorParamsAs1DForOutWhenUnconnected=off
  wires:
  Init/1 -> Switch/3
  Step/1 -> Switch/2
  Switch/1 -> Mean/1
  Gain/1 -> Switch/1
  Sum/1 -> Gain/1
  In/1 -> integrator/1
  integrator/1 -> Sum/1, Transport Delay/1
  Transport Delay/1 -> Sum/2

== system DFIG_FILTER/MODEL (PHASER)/Wind turbine Data acquisition1/magnitude positive seq.  ==
  In1 : Inport
  Complex to Real-Imag : ComplexToRealImag
  Fourier1 : Subsystem  mask(Fourier analyser){f1=60, n=0}
      mask prompts: f1 "Fundamental frequency f1 (Hz):"; n "Harmonic n (0=DC; 1=fundamental; 2=2nd harm;  ...) :"
      mask help: The Fourier block performs a Fourier analysis of the input signal over a running window of one cycle of the fundamental frequency. First and second outputs return respectively the magnitude and phase (degrees) of the harmonic component specified.
      mask init:
      | k=2-(n==0);
      mask Help: helpview(psbhelp)
  Fourier2 : Subsystem  mask(Fourier analyser){f1=60, n=0}
      mask prompts: f1 "Fundamental frequency f1 (Hz):"; n "Harmonic n (0=DC; 1=fundamental; 2=2nd harm;  ...) :"
      mask help: The Fourier block performs a Fourier analysis of the input signal over a running window of one cycle of the fundamental frequency. First and second outputs return respectively the magnitude and phase (degrees) of the harmonic component specified.
      mask init:
      | k=2-(n==0);
      mask Help: helpview(psbhelp)
  Math Function : Math  Operator=hypot  SignedPower=on
  Terminator : Terminator
  Terminator1 : Terminator
  Out1 : Outport  VectorParamsAs1DForOutWhenUnconnected=off
  wires:
  In1/1 -> Complex to Real-Imag/1
  Math Function/1 -> Out1/1
  Fourier2/1(magnitude) -> Math Function/2
  Fourier1/1(magnitude) -> Math Function/1
  Fourier2/2(angle) -> Terminator1/1
  Fourier1/2(angle) -> Terminator/1
  Complex to Real-Imag/2 -> Fourier2/1(signal)
  Complex to Real-Imag/1 -> Fourier1/1(signal)

== system DFIG_FILTER/MODEL (PHASER)/Wind turbine Data acquisition1/magnitude positivie seq ==
  In1 : Inport
  Complex to Real-Imag : ComplexToRealImag
  Fourier1 : Subsystem  mask(Fourier analyser){f1=60, n=0}
      mask prompts: f1 "Fundamental frequency f1 (Hz):"; n "Harmonic n (0=DC; 1=fundamental; 2=2nd harm;  ...) :"
      mask help: The Fourier block performs a Fourier analysis of the input signal over a running window of one cycle of the fundamental frequency. First and second outputs return respectively the magnitude and phase (degrees) of the harmonic component specified.
      mask init:
      | k=2-(n==0);
      mask Help: helpview(psbhelp)
  Fourier2 : Subsystem  mask(Fourier analyser){f1=60, n=0}
      mask prompts: f1 "Fundamental frequency f1 (Hz):"; n "Harmonic n (0=DC; 1=fundamental; 2=2nd harm;  ...) :"
      mask help: The Fourier block performs a Fourier analysis of the input signal over a running window of one cycle of the fundamental frequency. First and second outputs return respectively the magnitude and phase (degrees) of the harmonic component specified.
      mask init:
      | k=2-(n==0);
      mask Help: helpview(psbhelp)
  Math Function : Math  Operator=hypot  SignedPower=on
  Terminator : Terminator
  Terminator1 : Terminator
  Out1 : Outport  VectorParamsAs1DForOutWhenUnconnected=off
  wires:
  Complex to Real-Imag/1 -> Fourier1/1(signal)
  Complex to Real-Imag/2 -> Fourier2/1(signal)
  Fourier1/2(angle) -> Terminator/1
  Fourier2/2(angle) -> Terminator1/1
  Fourier1/1(magnitude) -> Math Function/1
  Fourier2/1(magnitude) -> Math Function/2
  Math Function/1 -> Out1/1
  In1/1 -> Complex to Real-Imag/1

== system DFIG_FILTER/MODEL (PHASER)/Wind turbine Data acquisition2/Mean Value1 ==
  note: Mean value
  In : Inport
  Init : Inport  Port=2
  Gain : Gain  Gain=1/Period  SaturateOnIntegerOverflow=on  OutDataTypeStr=Inherit: Same as input  ParamDataTypeStr=Inherit: Same as input
  Step : Step  Time=Period+eps  SampleTime=0
  Sum : Sum  Inputs=+-  InputSameDT=on  SaturateOnIntegerOverflow=on  OutDataTypeStr=Inherit: Same as first input
  Switch : Switch  Threshold=0.5  InputSameDT=off
  Transport Delay : TransportDelay  DelayTime=Period
  integrator : Integrator
  Mean : Outport  VectorParamsAs1DForOutWhenUnconnected=off
  wires:
  Transport Delay/1 -> Sum/2
  integrator/1 -> Transport Delay/1, Sum/1
  In/1 -> integrator/1
  Sum/1 -> Gain/1
  Gain/1 -> Switch/1
  Switch/1 -> Mean/1
  Step/1 -> Switch/2
  Init/1 -> Switch/3

== system DFIG_FILTER/MODEL (PHASER)/Wind turbine Data acquisition2/Mean Value2 ==
  note: Mean value
  In : Inport
  Init : Inport  Port=2
  Gain : Gain  Gain=1/Period  SaturateOnIntegerOverflow=on  OutDataTypeStr=Inherit: Same as input  ParamDataTypeStr=Inherit: Same as input
  Step : Step  Time=Period+eps  SampleTime=0
  Sum : Sum  Inputs=+-  InputSameDT=on  SaturateOnIntegerOverflow=on  OutDataTypeStr=Inherit: Same as first input
  Switch : Switch  Threshold=0.5  InputSameDT=off
  Transport Delay : TransportDelay  DelayTime=Period
  integrator : Integrator
  Mean : Outport  VectorParamsAs1DForOutWhenUnconnected=off
  wires:
  Init/1 -> Switch/3
  Step/1 -> Switch/2
  Switch/1 -> Mean/1
  Gain/1 -> Switch/1
  Sum/1 -> Gain/1
  In/1 -> integrator/1
  integrator/1 -> Sum/1, Transport Delay/1
  Transport Delay/1 -> Sum/2

== system DFIG_FILTER/MODEL (PHASER)/Wind turbine Data acquisition2/magnitude positive seq.  ==
  In1 : Inport
  Complex to Real-Imag : ComplexToRealImag
  Fourier1 : Subsystem  mask(Fourier analyser){f1=60, n=0}
      mask prompts: f1 "Fundamental frequency f1 (Hz):"; n "Harmonic n (0=DC; 1=fundamental; 2=2nd harm;  ...) :"
      mask help: The Fourier block performs a Fourier analysis of the input signal over a running window of one cycle of the fundamental frequency. First and second outputs return respectively the magnitude and phase (degrees) of the harmonic component specified.
      mask init:
      | k=2-(n==0);
      mask Help: helpview(psbhelp)
  Fourier2 : Subsystem  mask(Fourier analyser){f1=60, n=0}
      mask prompts: f1 "Fundamental frequency f1 (Hz):"; n "Harmonic n (0=DC; 1=fundamental; 2=2nd harm;  ...) :"
      mask help: The Fourier block performs a Fourier analysis of the input signal over a running window of one cycle of the fundamental frequency. First and second outputs return respectively the magnitude and phase (degrees) of the harmonic component specified.
      mask init:
      | k=2-(n==0);
      mask Help: helpview(psbhelp)
  Math Function : Math  Operator=hypot  SignedPower=on
  Terminator : Terminator
  Terminator1 : Terminator
  Out1 : Outport  VectorParamsAs1DForOutWhenUnconnected=off
  wires:
  In1/1 -> Complex to Real-Imag/1
  Math Function/1 -> Out1/1
  Fourier2/1(magnitude) -> Math Function/2
  Fourier1/1(magnitude) -> Math Function/1
  Fourier2/2(angle) -> Terminator1/1
  Fourier1/2(angle) -> Terminator/1
  Complex to Real-Imag/2 -> Fourier2/1(signal)
  Complex to Real-Imag/1 -> Fourier1/1(signal)

== system DFIG_FILTER/MODEL (PHASER)/Wind turbine Data acquisition2/magnitude positivie seq ==
  In1 : Inport
  Complex to Real-Imag : ComplexToRealImag
  Fourier1 : Subsystem  mask(Fourier analyser){f1=60, n=0}
      mask prompts: f1 "Fundamental frequency f1 (Hz):"; n "Harmonic n (0=DC; 1=fundamental; 2=2nd harm;  ...) :"
      mask help: The Fourier block performs a Fourier analysis of the input signal over a running window of one cycle of the fundamental frequency. First and second outputs return respectively the magnitude and phase (degrees) of the harmonic component specified.
      mask init:
      | k=2-(n==0);
      mask Help: helpview(psbhelp)
  Fourier2 : Subsystem  mask(Fourier analyser){f1=60, n=0}
      mask prompts: f1 "Fundamental frequency f1 (Hz):"; n "Harmonic n (0=DC; 1=fundamental; 2=2nd harm;  ...) :"
      mask help: The Fourier block performs a Fourier analysis of the input signal over a running window of one cycle of the fundamental frequency. First and second outputs return respectively the magnitude and phase (degrees) of the harmonic component specified.
      mask init:
      | k=2-(n==0);
      mask Help: helpview(psbhelp)
  Math Function : Math  Operator=hypot  SignedPower=on
  Terminator : Terminator
  Terminator1 : Terminator
  Out1 : Outport  VectorParamsAs1DForOutWhenUnconnected=off
  wires:
  Complex to Real-Imag/1 -> Fourier1/1(signal)
  Complex to Real-Imag/2 -> Fourier2/1(signal)
  Fourier1/2(angle) -> Terminator/1
  Fourier2/2(angle) -> Terminator1/1
  Fourier1/1(magnitude) -> Math Function/1
  Fourier2/1(magnitude) -> Math Function/2
  Math Function/1 -> Out1/1
  In1/1 -> Complex to Real-Imag/1

== system DFIG_FILTER/MODEL (PHASER)/Wind turbine Data acquisition3/Mean Value1 ==
  note: Mean value
  In : Inport
  Init : Inport  Port=2
  Gain : Gain  Gain=1/Period  SaturateOnIntegerOverflow=on  OutDataTypeStr=Inherit: Same as input  ParamDataTypeStr=Inherit: Same as input
  Step : Step  Time=Period+eps  SampleTime=0
  Sum : Sum  Inputs=+-  InputSameDT=on  SaturateOnIntegerOverflow=on  OutDataTypeStr=Inherit: Same as first input
  Switch : Switch  Threshold=0.5  InputSameDT=off
  Transport Delay : TransportDelay  DelayTime=Period
  integrator : Integrator
  Mean : Outport  VectorParamsAs1DForOutWhenUnconnected=off
  wires:
  Transport Delay/1 -> Sum/2
  integrator/1 -> Transport Delay/1, Sum/1
  In/1 -> integrator/1
  Sum/1 -> Gain/1
  Gain/1 -> Switch/1
  Switch/1 -> Mean/1
  Step/1 -> Switch/2
  Init/1 -> Switch/3

== system DFIG_FILTER/MODEL (PHASER)/Wind turbine Data acquisition3/Mean Value2 ==
  note: Mean value
  In : Inport
  Init : Inport  Port=2
  Gain : Gain  Gain=1/Period  SaturateOnIntegerOverflow=on  OutDataTypeStr=Inherit: Same as input  ParamDataTypeStr=Inherit: Same as input
  Step : Step  Time=Period+eps  SampleTime=0
  Sum : Sum  Inputs=+-  InputSameDT=on  SaturateOnIntegerOverflow=on  OutDataTypeStr=Inherit: Same as first input
  Switch : Switch  Threshold=0.5  InputSameDT=off
  Transport Delay : TransportDelay  DelayTime=Period
  integrator : Integrator
  Mean : Outport  VectorParamsAs1DForOutWhenUnconnected=off
  wires:
  Init/1 -> Switch/3
  Step/1 -> Switch/2
  Switch/1 -> Mean/1
  Gain/1 -> Switch/1
  Sum/1 -> Gain/1
  In/1 -> integrator/1
  integrator/1 -> Sum/1, Transport Delay/1
  Transport Delay/1 -> Sum/2

== system DFIG_FILTER/MODEL (PHASER)/Wind turbine Data acquisition3/magnitude positive seq.  ==
  In1 : Inport
  Complex to Real-Imag : ComplexToRealImag
  Fourier1 : Subsystem  mask(Fourier analyser){f1=60, n=0}
      mask prompts: f1 "Fundamental frequency f1 (Hz):"; n "Harmonic n (0=DC; 1=fundamental; 2=2nd harm;  ...) :"
      mask help: The Fourier block performs a Fourier analysis of the input signal over a running window of one cycle of the fundamental frequency. First and second outputs return respectively the magnitude and phase (degrees) of the harmonic component specified.
      mask init:
      | k=2-(n==0);
      mask Help: helpview(psbhelp)
  Fourier2 : Subsystem  mask(Fourier analyser){f1=60, n=0}
      mask prompts: f1 "Fundamental frequency f1 (Hz):"; n "Harmonic n (0=DC; 1=fundamental; 2=2nd harm;  ...) :"
      mask help: The Fourier block performs a Fourier analysis of the input signal over a running window of one cycle of the fundamental frequency. First and second outputs return respectively the magnitude and phase (degrees) of the harmonic component specified.
      mask init:
      | k=2-(n==0);
      mask Help: helpview(psbhelp)
  Math Function : Math  Operator=hypot  SignedPower=on
  Terminator : Terminator
  Terminator1 : Terminator
  Out1 : Outport  VectorParamsAs1DForOutWhenUnconnected=off
  wires:
  In1/1 -> Complex to Real-Imag/1
  Math Function/1 -> Out1/1
  Fourier2/1(magnitude) -> Math Function/2
  Fourier1/1(magnitude) -> Math Function/1
  Fourier2/2(angle) -> Terminator1/1
  Fourier1/2(angle) -> Terminator/1
  Complex to Real-Imag/2 -> Fourier2/1(signal)
  Complex to Real-Imag/1 -> Fourier1/1(signal)

== system DFIG_FILTER/MODEL (PHASER)/Wind turbine Data acquisition3/magnitude positivie seq ==
  In1 : Inport
  Complex to Real-Imag : ComplexToRealImag
  Fourier1 : Subsystem  mask(Fourier analyser){f1=60, n=0}
      mask prompts: f1 "Fundamental frequency f1 (Hz):"; n "Harmonic n (0=DC; 1=fundamental; 2=2nd harm;  ...) :"
      mask help: The Fourier block performs a Fourier analysis of the input signal over a running window of one cycle of the fundamental frequency. First and second outputs return respectively the magnitude and phase (degrees) of the harmonic component specified.
      mask init:
      | k=2-(n==0);
      mask Help: helpview(psbhelp)
  Fourier2 : Subsystem  mask(Fourier analyser){f1=60, n=0}
      mask prompts: f1 "Fundamental frequency f1 (Hz):"; n "Harmonic n (0=DC; 1=fundamental; 2=2nd harm;  ...) :"
      mask help: The Fourier block performs a Fourier analysis of the input signal over a running window of one cycle of the fundamental frequency. First and second outputs return respectively the magnitude and phase (degrees) of the harmonic component specified.
      mask init:
      | k=2-(n==0);
      mask Help: helpview(psbhelp)
  Math Function : Math  Operator=hypot  SignedPower=on
  Terminator : Terminator
  Terminator1 : Terminator
  Out1 : Outport  VectorParamsAs1DForOutWhenUnconnected=off
  wires:
  Complex to Real-Imag/1 -> Fourier1/1(signal)
  Complex to Real-Imag/2 -> Fourier2/1(signal)
  Fourier1/2(angle) -> Terminator/1
  Fourier2/2(angle) -> Terminator1/1
  Fourier1/1(magnitude) -> Math Function/1
  Fourier2/1(magnitude) -> Math Function/2
  Math Function/1 -> Out1/1
  In1/1 -> Complex to Real-Imag/1

== system DFIG_FILTER/MODEL (PHASER)/Wind turbine Data acquisition4/Mean Value1 ==
  note: Mean value
  In : Inport
  Init : Inport  Port=2
  Gain : Gain  Gain=1/Period  SaturateOnIntegerOverflow=on  OutDataTypeStr=Inherit: Same as input  ParamDataTypeStr=Inherit: Same as input
  Step : Step  Time=Period+eps  SampleTime=0
  Sum : Sum  Inputs=+-  InputSameDT=on  SaturateOnIntegerOverflow=on  OutDataTypeStr=Inherit: Same as first input
  Switch : Switch  Threshold=0.5  InputSameDT=off
  Transport Delay : TransportDelay  DelayTime=Period
  integrator : Integrator
  Mean : Outport  VectorParamsAs1DForOutWhenUnconnected=off
  wires:
  Transport Delay/1 -> Sum/2
  integrator/1 -> Transport Delay/1, Sum/1
  In/1 -> integrator/1
  Sum/1 -> Gain/1
  Gain/1 -> Switch/1
  Switch/1 -> Mean/1
  Step/1 -> Switch/2
  Init/1 -> Switch/3
